simulink model "Rebuilt_AWD"  (R2022a)
settings: Solver=VariableStepAuto  StartTime=0.0  StopTime=100  MaxStep=0.01  RelTol=1e-3
PreLoadFcn:
  | open Vehicle_information
  | run  Vehicle_information
undefined symbols (not defined in the file or in its folder): Rider_mass, sigbuilder_block, Vehicle_mass, wheel_radius
libraries: nesl_utility x30, fl_lib x26, sdl_lib x19
(part 1 of 3)
CloseFcn:
  | clc
  | clear
settings Model: Creator=Aqib Habib  LastModifiedBy=Aqib Habib
settings SolverCC: AlgebraicLoopSolver=LineSearch
settings DebuggingCC: UnconnectedInputMsg=warning  UnconnectedOutputMsg=warning  UnconnectedLineMsg=warning  SFMachineParentedDataDiag=warning
settings SFSimCC: CustomCodeUndefinedFunction=UseInterfaceOnly

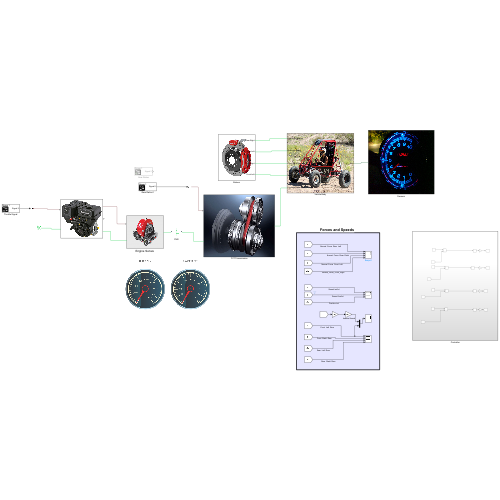
[thumbnail: Simulink's stored preview of the top-level diagram]
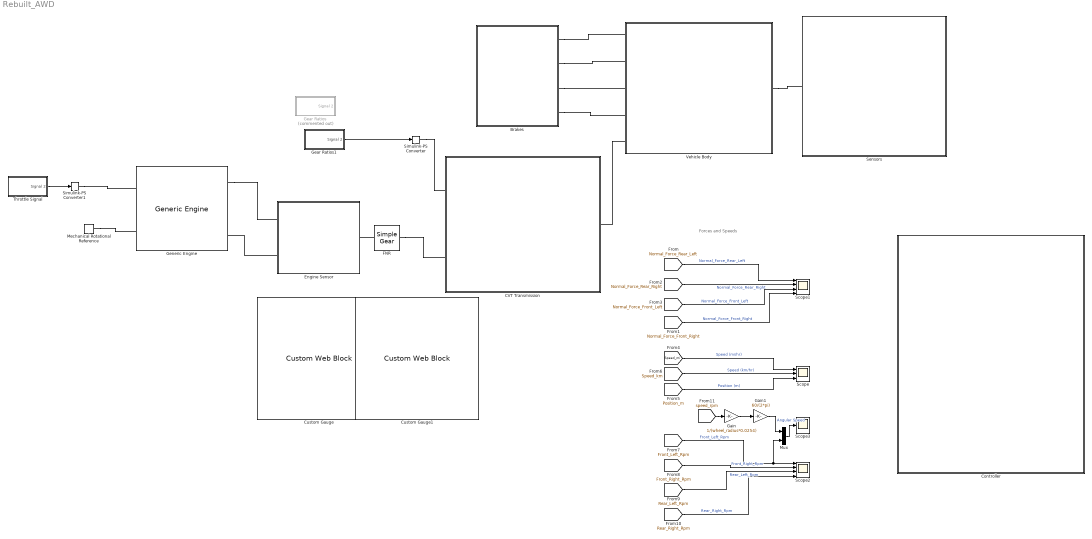
== system Rebuilt_AWD ==
  note: Forces and Speeds
  Brakes : Subsystem
      mask Display: image('brake_kit_140-14883-DR-xl.jpg');
  CVT Transmission : Subsystem
      mask Display: image('CVT-58e526803df78c5162b323c9.jpg');
  "Controller " : Subsystem
  Custom Gauge : CustomWebBlock  Configuration="{\"components\":[{\"name\":\"CircularScaleComponent\",\"settings\":{\"bounds\":{\"max\":100,\"min\":0,\"tickInterval\":\"auto\"},\"direction\":\"cw\",\"flipLimits\":0,\"innerRadius\":0.75,\"internalTickHeightScaleFactor\":1,\"labelColor\":[255,252,199],\"labelFont\":{\"font\":\"Arial\",\"fontSize\":12},\"labelRadius\":0.36,\"labelTransparency\":1,\"minorTickHeightScaleFactor\":0.2,\"needleImage\":{\"size\":[1890,567],\"src\":\"data:image\\/svg+xml;base64,PD94bWwgdmVyc2lvbj0iMS4wIiBlbmNvZGluZz0iVVRGLTgiIHN0YW5kYWxvbmU9Im5vIj8+CjxzdmcKICAgeG1sbnM6ZGM9Imh0dHA6Ly9wdXJsLm9yZy9kYy9lbGVtZW50cy8xLjEvIgogICB4bWxuczpjYz0iaHR0cDovL2NyZWF0aXZlY29tbW9ucy5vcmcvbnMjIgogICB4bWxuczpyZGY9Imh0dHA6Ly93d3cudzMub3JnLzE5OTkvMDIvMjItcmRmLXN5bnRheC1ucyMiCiAgIHhtbG5zOnN2Zz0iaHR0cDovL3d3dy53My5vcmcvMjAwMC9zdmciCiAgIHhtbG5zPSJodHRwOi8vd3d3LnczLm9yZy8yMDAwL3N2ZyIKICAgeG1sbnM6 ...(+4096 chars)\"},\"needleOffset\":[0.14,0],\"needleOrientation\":-45,\"needleRotation\":180,\"needleSize\":{\"height\":0.13,\"width\":0.41},\"outerRadius\":0.9,\"position\":[0.06486742424242424,0.05627705627705628,0.8917748917748918,0.8787878787878788],\"scaleAngle\":270,\"scaleAngleOffset\":135,\"scaleColors\":[],\"scaleColorsSize\":0.2,\"scalePosition\":[0,0,1,1],\"showLabels\":1,\"showMinorTicks\":1,\"showSpanLine\":1,\"showTicks\":1,\"tickColor\":[255,255,200],\"tickTransparency\":1,\"valueBarColor\":[0,114,189],\"valueBarPosition\":[0,0,1,1],\"valueBarSize\":0.2,\"valueBarTransparency\":1}},{\"name\":\"BackgroundImageComponent\",\"settings\":{\"image\":{\"size\":[500,500],\"src\":\"data:image\\/svg+xml;base64,PD94bWwgdmVyc2lvbj0iMS4wIiBlbmNvZGluZz0iVVRGLTgiIHN0YW5kYWxvbmU9Im5vIj8+CjxzdmcKICAgeG1sbnM6ZGM9Imh0dHA6Ly9wdXJsLm9yZy9kYy9lbGVtZW50cy8xLjEvIgogICB4bWxuczpjYz0iaHR0cDovL2NyZWF0aXZlY29tbW9ucy5vcmcvbnMjIgogICB4bWxuczpyZGY9Imh0dHA6Ly93d3cudzMub3JnLzE5OTkvMDIvMjItcmRmLXN5bnRheC1ucyMiCiAgIHhtbG5zOnN2Zz0iaHR0cDovL3d3dy53My5vcmcvMjAwMC9zdmciCiAgIHhtbG5zPSJodHRwOi8vd3d3LnczLm9yZy8yMDAwL3N2ZyIKICAgeG1sbnM6 ...(+9964 chars)\"},\"position\":[0,0,1,1],\"scaleMode\":\"0\"}},{\"name\":\"ForegroundImageComponent\",\"settings\":{\"image\":{\"size\":[0,0],\"src\":\"default\",\"srcOrientation\":[]},\"isForeground\":1,\"position\":[0,0,1,1],\"scaleMode\":\"0\"}}],\"legacySettings\":{\"BackgroundImage\":\"data:image\\/svg+xml;base64,PD94bWwgdmVyc2lvbj0iMS4wIiBlbmNvZGluZz0iVVRGLTgiIHN0YW5kYWxvbmU9Im5vIj8+CjwhLS0gR2VuZXJhdG9yOiBBZG9iZSBJbGx1c3RyYXRvciAxOS4yLjEsIFNWRyBFeHBvcnQgUGx1Zy1JbiAuIFNWRyBWZXJzaW9uOiA2LjAwIEJ1aWxkIDApICAtLT4KCjxzdmcKICAgeG1sbnM6ZGM9Imh0dHA6Ly9wdXJsLm9yZy9kYy9lbGVtZW50cy8xLjEvIgogICB4bWxuczpjYz0iaHR0cDovL2NyZWF0aXZlY29tbW9ucy5vcmcvbnMjIgogICB4bWxuczpyZGY9Imh0dHA6Ly93d3cudzMub3JnLzE5OTkvMDIvMjItcmRmLXN5bnRh ...(+9660 chars)\",\"CenterOffsetX\":\"0\",\"CenterOffsetY\":\"0\",\"GaugeArcColor\":\"#9ec0f7\",\"GaugeArcDefined\":\"true\",\"GaugeArcRadius\":\"0.1358563990074277\",\"GaugeArcRatio\":\"0.8333333333333\",\"GaugeArcRotation\":\"240.5385250290321\",\"GaugeArcStrokeWidth\":\"0.03972965542329953\",\"GaugeArcTransparency\":\"0\",\"GaugeMax\":\"3800\",\"GaugeMin\":\"0\",\"GaugeTickColor\":\"#faf5c8\",\"GaugeTickTransparency\":\"1\",\"GaugeTickVisible\":\"true\",\"GaugeValue\":\"0\",\"NeedleHeight\":\"0.11602152693163792\",\"NeedleImage\":\"data:image\\/svg+xml;base64,PD94bWwgdmVyc2lvbj0iMS4wIiBlbmNvZGluZz0idXRmLTgiPz4KPCEtLSBHZW5lcmF0b3I6IEFkb2JlIElsbHVzdHJhdG9yIDE5LjIuMSwgU1ZHIEV4cG9ydCBQbHVnLUluIC4gU1ZHIFZlcnNpb246IDYuMDAgQnVpbGQgMCkgIC0tPgo8c3ZnIHZlcnNpb249IjEuMSIgeG1sbnM9Imh0dHA6Ly93d3cudzMub3JnLzIwMDAvc3ZnIiB4bWxuczp4bGluaz0iaHR0cDovL3d3dy53My5vcmcvMTk5OS94bGluayIgeD0iMHB4IiB5PSIwcHgiCgkgdmlld0JveD0iMCAwIDIwMCA1MCIgc3R5bGU9ImVuYWJsZS1iYWNrZ3JvdW5kOm5ldyAw ...(+9940 chars)\",\"NeedleInitialRotation\":\"-59.94322499147643\",\"NeedleWidth\":\"0.1911368983686954\",\"NeedleXPos\":\"0.3802298124325669\",\"NeedleYPos\":\"0.48117305677424654\",\"ScaleColorsJSON\":\"[]\",\"ValueArcColor\":\"#1759b0\",\"ValueArcTransparency\":\"1\"},\"settings\":{\"BindingType\":\"signal\",\"backgroundOffset\":0.14,\"backgroundOpacity\":1,\"fixedAspectRatio\":\"on\",\"showBackgroundColor\":0},\"type\":\"CircularGauge\"}"
  Custom Gauge1 : CustomWebBlock  Configuration="{\"components\":[{\"name\":\"CircularScaleComponent\",\"settings\":{\"bounds\":{\"max\":100,\"min\":0,\"tickInterval\":\"auto\"},\"direction\":\"cw\",\"flipLimits\":0,\"innerRadius\":0.75,\"internalTickHeightScaleFactor\":1,\"labelColor\":[255,252,199],\"labelFont\":{\"font\":\"Arial\",\"fontSize\":12},\"labelRadius\":0.36,\"labelTransparency\":1,\"minorTickHeightScaleFactor\":0.2,\"needleImage\":{\"size\":[1890,567],\"src\":\"data:image\\/svg+xml;base64,PD94bWwgdmVyc2lvbj0iMS4wIiBlbmNvZGluZz0iVVRGLTgiIHN0YW5kYWxvbmU9Im5vIj8+CjxzdmcKICAgeG1sbnM6ZGM9Imh0dHA6Ly9wdXJsLm9yZy9kYy9lbGVtZW50cy8xLjEvIgogICB4bWxuczpjYz0iaHR0cDovL2NyZWF0aXZlY29tbW9ucy5vcmcvbnMjIgogICB4bWxuczpyZGY9Imh0dHA6Ly93d3cudzMub3JnLzE5OTkvMDIvMjItcmRmLXN5bnRheC1ucyMiCiAgIHhtbG5zOnN2Zz0iaHR0cDovL3d3dy53My5vcmcvMjAwMC9zdmciCiAgIHhtbG5zPSJodHRwOi8vd3d3LnczLm9yZy8yMDAwL3N2ZyIKICAgeG1sbnM6 ...(+4096 chars)\"},\"needleOffset\":[0.14,0],\"needleOrientation\":-45,\"needleRotation\":180,\"needleSize\":{\"height\":0.13,\"width\":0.41},\"outerRadius\":0.9,\"position\":[0.06486742424242424,0.05627705627705628,0.8917748917748918,0.8787878787878788],\"scaleAngle\":270,\"scaleAngleOffset\":135,\"scaleColors\":[],\"scaleColorsSize\":0.2,\"scalePosition\":[0,0,1,1],\"showLabels\":1,\"showMinorTicks\":1,\"showSpanLine\":1,\"showTicks\":1,\"tickColor\":[255,255,200],\"tickTransparency\":1,\"valueBarColor\":[0,114,189],\"valueBarPosition\":[0,0,1,1],\"valueBarSize\":0.2,\"valueBarTransparency\":1}},{\"name\":\"BackgroundImageComponent\",\"settings\":{\"image\":{\"size\":[500,500],\"src\":\"data:image\\/svg+xml;base64,PD94bWwgdmVyc2lvbj0iMS4wIiBlbmNvZGluZz0iVVRGLTgiIHN0YW5kYWxvbmU9Im5vIj8+CjxzdmcKICAgeG1sbnM6ZGM9Imh0dHA6Ly9wdXJsLm9yZy9kYy9lbGVtZW50cy8xLjEvIgogICB4bWxuczpjYz0iaHR0cDovL2NyZWF0aXZlY29tbW9ucy5vcmcvbnMjIgogICB4bWxuczpyZGY9Imh0dHA6Ly93d3cudzMub3JnLzE5OTkvMDIvMjItcmRmLXN5bnRheC1ucyMiCiAgIHhtbG5zOnN2Zz0iaHR0cDovL3d3dy53My5vcmcvMjAwMC9zdmciCiAgIHhtbG5zPSJodHRwOi8vd3d3LnczLm9yZy8yMDAwL3N2ZyIKICAgeG1sbnM6 ...(+9964 chars)\"},\"position\":[0,0,1,1],\"scaleMode\":\"0\"}},{\"name\":\"ForegroundImageComponent\",\"settings\":{\"image\":{\"size\":[0,0],\"src\":\"default\",\"srcOrientation\":[]},\"isForeground\":1,\"position\":[0,0,1,1],\"scaleMode\":\"0\"}}],\"legacySettings\":{\"BackgroundImage\":\"data:image\\/svg+xml;base64,PD94bWwgdmVyc2lvbj0iMS4wIiBlbmNvZGluZz0iVVRGLTgiIHN0YW5kYWxvbmU9Im5vIj8+CjwhLS0gR2VuZXJhdG9yOiBBZG9iZSBJbGx1c3RyYXRvciAxOS4yLjEsIFNWRyBFeHBvcnQgUGx1Zy1JbiAuIFNWRyBWZXJzaW9uOiA2LjAwIEJ1aWxkIDApICAtLT4KCjxzdmcKICAgeG1sbnM6ZGM9Imh0dHA6Ly9wdXJsLm9yZy9kYy9lbGVtZW50cy8xLjEvIgogICB4bWxuczpjYz0iaHR0cDovL2NyZWF0aXZlY29tbW9ucy5vcmcvbnMjIgogICB4bWxuczpyZGY9Imh0dHA6Ly93d3cudzMub3JnLzE5OTkvMDIvMjItcmRmLXN5bnRh ...(+9660 chars)\",\"CenterOffsetX\":\"0\",\"CenterOffsetY\":\"0\",\"GaugeArcColor\":\"#9ec0f7\",\"GaugeArcDefined\":\"true\",\"GaugeArcRadius\":\"0.1358563990074277\",\"GaugeArcRatio\":\"0.8333333333333\",\"GaugeArcRotation\":\"240.5385250290321\",\"GaugeArcStrokeWidth\":\"0.03972965542329953\",\"GaugeArcTransparency\":\"0\",\"GaugeMax\":\"100\",\"GaugeMin\":\"0\",\"GaugeTickColor\":\"#faf5c8\",\"GaugeTickTransparency\":\"1\",\"GaugeTickVisible\":\"true\",\"GaugeValue\":\"0\",\"NeedleHeight\":\"0.11602152693163792\",\"NeedleImage\":\"data:image\\/svg+xml;base64,PD94bWwgdmVyc2lvbj0iMS4wIiBlbmNvZGluZz0idXRmLTgiPz4KPCEtLSBHZW5lcmF0b3I6IEFkb2JlIElsbHVzdHJhdG9yIDE5LjIuMSwgU1ZHIEV4cG9ydCBQbHVnLUluIC4gU1ZHIFZlcnNpb246IDYuMDAgQnVpbGQgMCkgIC0tPgo8c3ZnIHZlcnNpb249IjEuMSIgeG1sbnM9Imh0dHA6Ly93d3cudzMub3JnLzIwMDAvc3ZnIiB4bWxuczp4bGluaz0iaHR0cDovL3d3dy53My5vcmcvMTk5OS94bGluayIgeD0iMHB4IiB5PSIwcHgiCgkgdmlld0JveD0iMCAwIDIwMCA1MCIgc3R5bGU9ImVuYWJsZS1iYWNrZ3JvdW5kOm5ldyAw ...(+9940 chars)\",\"NeedleInitialRotation\":\"-59.94322499147643\",\"NeedleWidth\":\"0.1911368983686954\",\"NeedleXPos\":\"0.3802298124325669\",\"NeedleYPos\":\"0.48117305677424654\",\"ScaleColorsJSON\":\"[]\",\"ValueArcColor\":\"#1759b0\",\"ValueArcTransparency\":\"1\"},\"settings\":{\"BindingType\":\"signal\",\"backgroundOffset\":0.14,\"backgroundOpacity\":1,\"fixedAspectRatio\":\"on\",\"showBackgroundColor\":0},\"type\":\"CircularGauge\"}"
  Engine Sensor : Subsystem
      mask Display: image('eddy-current-engine-dynamometer_cat-1024x878.jpg');
  FNR : sdl_lib/Gears/Simple Gear  ratio=4  rotation_direction=3-2*(1)  friction_model=sdl.enum.gear_efficiencies_load.off  T_noload=0.1 N*m  T_nom=5 N*m  efficiency_nom=0.8  efficiency=0.8  temperature_TLU=[280, 300, 320] K  load_TLU=[1, 5, 10] N*m  efficiency_TLU=[.95, .9, .85]  efficiency_TLU2=[.85, .8, .75; .95, .9, .85; .85, .8, .7]  w_thr=0.01 rad/s  pwr_thr=0.001 W  backlash_model=sdl.enum.backlashModel.Off  backlash_distance=1e-3 mm  x0=0 mm  r_base=0.1 m  hardstop_model=simscape.enum.hardstop.smooth  transition=1e-4 mm  backlash_stiffness=1e7 N/m  backlash_damping=1e6 N*s/m  e=0  v_tol=0.001 m/s  mu_visc=[0, 0] N*m/(rad/s)  enable_faults=simscape.enum.onoff.off  efficiency_fault=0.05  external_fault=simscape.enum.onoff.off  temporal_fault=simscape.enum.onoff.off  fault_time=5 s  fault_angles=pi / 12 rad  report_fault=(1)-1  thermal_mass=50 J/K  temperature_specify=off  temperature_priority=High  temperature=300 K  temperature_nominal_specify=off  temperature_nominal_unit=K  temperature_nominal_value=1  x_backlash_specify=off  x_backlash_priority=None  x_backlash=0 mm  x_backlash_nominal_specify=off  x_backlash_nominal_unit=mm  x_backlash_nominal_value=1  f_hardstop_specify=off  f_hardstop_priority=None  f_hardstop=0 N  f_hardstop_nominal_specify=off  f_hardstop_nominal_unit=N  f_hardstop_nominal_value=1  v_backlash_specify=off  v_backlash_priority=None  v_backlash=0 m/s  v_backlash_nominal_specify=off  v_backlash_nominal_unit=m/s  v_backlash_nominal_value=1
  Gain : Gain  Gain=1/(wheel_radius*0.0254)
  Gain1 : Gain  Gain=60/(2*pi)
  Gear Ratios : Subsystem  Tag=STV Subsys  Commented=on  LoadFcn=sigbuilder_block('load');  StartFcn=sigbuilder_block('start');  StopFcn=sigbuilder_block('stop');  ClipboardFcn=sigbuilder_block('clipboard');  mask(Sigbuilder block){tuvar=[0:10]}
      mask help: Simulink:masks:SigbuilderBlock_MD
      mask init:
      | if ~strcmp(get_param(bdroot(gcbh),'SimulationStatus'),'stopped') tuvar = sigbuilder_block('maskInit'); end
      settings: CopyFcn=sigbuilder_block('copy');  DeleteFcn=sigbuilder_block('delete');  ModelCloseFcn=sigbuilder_block('modelClose');  PreSaveFcn=sigbuilder_block('preSave');  PauseFcn=sigbuilder_block('pause');  ContinueFcn=sigbuilder_block('continue');  NameChangeFcn=sigbuilder_block('namechange');  OpenFcn=sigbuilder_block('open',[6 30 1428 681.75 ]);  CloseFcn=sigbuilder_block('close');
      mask Display: plot(0, 0, 100, 100,[2, 2, 32, 32, 2], [68, 8, 8, 68, 68],[32, 2], [38, 38], [32, 19, 2],[53, 60, 44], [32, 17, 17, 2],[16, 16, 31, 31]);txt = getActiveGroup(gcbh);text(2, 100, txt,'verticalAlignment', 'top');
  Gear Ratios1 : Subsystem  Tag=STV Subsys  LoadFcn=sigbuilder_block('load');  StartFcn=sigbuilder_block('start');  StopFcn=sigbuilder_block('stop');  ClipboardFcn=sigbuilder_block('clipboard');  mask(Sigbuilder block){tuvar=[0:10]}
      mask help: Simulink:masks:SigbuilderBlock_MD
      mask init:
      | if ~strcmp(get_param(bdroot(gcbh),'SimulationStatus'),'stopped') tuvar = sigbuilder_block('maskInit'); end
      settings: CopyFcn=sigbuilder_block('copy');  DeleteFcn=sigbuilder_block('delete');  ModelCloseFcn=sigbuilder_block('modelClose');  PreSaveFcn=sigbuilder_block('preSave');  PauseFcn=sigbuilder_block('pause');  ContinueFcn=sigbuilder_block('continue');  NameChangeFcn=sigbuilder_block('namechange');  OpenFcn=sigbuilder_block('open',[6 30 1428 681.75 ]);  CloseFcn=sigbuilder_block('close');
      mask Display: plot(0, 0, 100, 100,[2, 2, 32, 32, 2], [68, 8, 8, 68, 68],[32, 2], [38, 38], [32, 19, 2],[53, 60, 44], [32, 17, 17, 2],[16, 16, 31, 31]);txt = getActiveGroup(gcbh);text(2, 100, txt,'verticalAlignment', 'top');
  Generic Engine : sdl_lib/Engines & Motors/Generic Engine  model_parameterization=3  engine_type=1  P_max=150 kW  w_P_max=4500 rpm  w_max=6000 rpm  w_min=500 rpm  w_tab=RPM rpm  trq_tab=[380, 380, 380, 380, 350, 280, 200, 80] N*m  pwr_tab=POWER HP_DIN  interp_method=simscape.enum.interpolation.smooth  model_inertia=1  inertia=5 kg*m^2  initial_velocity=2200 rpm  model_time_constant=0  time_constant=0.2 s  T0=0  w_thr=100 rpm  fc_model=0  fc_per_rev=25 mg/rev  fc_w_tab=[1000, 2000, 3000, 4000, 5000, 6000] rpm  fc_trq_tab=[0, 80, 160, 200, 240, 320, 360, 400] N*m  fc_tab=[.5, .9, 1.4, 1.6, 1.9, 2.7, 3.4, 4.4; 1, 1.7, 2.7, 3.1, 3.6, 5, 6, 7.4; 1.4, 2.7, 4, 4.8, 5.6, 7.5, 8.5, 10.5; 2, 3.6, 5.8, 6.7, 8, 10.4, 11.7, 13.3; 2.5, 4.8, 7.9, 9.4, 10.8, 14, 16.2, 18.6; 3.1, 6, 10.3, 11.9, 13.8, 18.4, 22, 26.5] g/s  bmep_tab=[0, 250, 500, 625, 750, 1000, 1150, 1250] kPa  bsfc_tab=[410, 380, 300, 280, 270, 290, 320, 380; 410, 370, 290, 270, 260, 270, 285, 320; 415, 380, 290, 275, 265, 270, 270, 300; 420, 390, 310, 290, 285, 280, 280, 285; 430, 410, 340, 320, 310, 300, 310, 320; 450, 430, 370, 340, 330, 330, 350, 380] g/hr/kW  fc_interp_method=simscape.enum.interpolation.linear  idle_speed=0  idle_speed_reference=3600 rpm  tau_controller=1 s  idle_w_thr=1 rpm  redline=0  redline_speed=5000 rpm  tau_redline=1 s  redline_w_thr=1 rpm  displaced_volume=400 cm^3  rev_per_cycle=2  mask(Generic Engine){}
      settings: SourceProductBaseCode=LD  InternalSimscapePortConfiguration="{\"Bottom\":[],\"Left\":[{\"id\":\"T\",\"label\":\"T\",\"type\":\"input\"},{\"id\":\"B\",\"label\":\"B\",\"type\":\"foundation.mechanical.rotational.rotational\"}],\"Right\":[{\"id\":\"P\",\"label\":\"P\",\"type\":\"output\"},{\"id\":\"FC\",\"label\":\"FC\",\"type\":\"output\"},{\"id\":\"F\",\"label\":\"F\",\"type\":\"foundation.mechanical.rotational.rotational\"}],\"Top\":[]}"
      mask Display: image('10.0hp_updated.jpg');
  Mechanical Rotational Reference : fl_lib/Mechanical/Rotational Elements/Mechanical Rotational Reference
      settings: SourceProductBaseCode=PW,SS,VE
  Mux : Mux  Inputs=2
  Scope : Scope  NumInputPorts=3
  Scope1 : Scope  NumInputPorts=4
  Scope2 : Scope  NumInputPorts=4
  Scope3 : Scope
  Sensors : Subsystem
      mask Display: image('wp6910276.jpg');
  Simulink-PS Converter : nesl_utility/Simulink-PS Converter  PhysicalDomain=network_engine_domain  SubClassName=ps_input  LeftPortType=input  RightPortType=output  PseudoPeriodic=off  Frequencies=[]  NoiseDistribution=none  NoiseParameters=[]  Unit=1  AffineConversion=off  FilteringAndDerivatives=provide  SimscapeFilterOrder=1  InputFilterTimeConstant=0.001  UdotUserProvided=0
      settings: SourceProductBaseCode=SS,PW,VE
  Simulink-PS Converter1 : nesl_utility/Simulink-PS Converter  PhysicalDomain=network_engine_domain  SubClassName=ps_input  LeftPortType=input  RightPortType=output  PseudoPeriodic=off  Frequencies=[]  NoiseDistribution=none  NoiseParameters=[]  Unit=1  AffineConversion=off  FilteringAndDerivatives=provide  SimscapeFilterOrder=1  InputFilterTimeConstant=0.001  UdotUserProvided=0
      settings: SourceProductBaseCode=SS,PW,VE
  Throttle Signal : Subsystem  Tag=STV Subsys  LoadFcn=sigbuilder_block('load');  StartFcn=sigbuilder_block('start');  StopFcn=sigbuilder_block('stop');  ClipboardFcn=sigbuilder_block('clipboard');  mask(Sigbuilder block){tuvar=[0:10]}
      mask help: Simulink:masks:SigbuilderBlock_MD
      mask init:
      | if ~strcmp(get_param(bdroot(gcbh),'SimulationStatus'),'stopped') tuvar = sigbuilder_block('maskInit'); end
      settings: CopyFcn=sigbuilder_block('copy');  DeleteFcn=sigbuilder_block('delete');  ModelCloseFcn=sigbuilder_block('modelClose');  PreSaveFcn=sigbuilder_block('preSave');  PauseFcn=sigbuilder_block('pause');  ContinueFcn=sigbuilder_block('continue');  NameChangeFcn=sigbuilder_block('namechange');  OpenFcn=sigbuilder_block('open',[6 30 1428 681.75 ]);  CloseFcn=sigbuilder_block('close');
      mask Display: plot(0, 0, 100, 100,[2, 2, 32, 32, 2], [68, 8, 8, 68, 68],[32, 2], [38, 38], [32, 19, 2],[53, 60, 44], [32, 17, 17, 2],[16, 16, 31, 31]);txt = getActiveGroup(gcbh);text(2, 100, txt,'verticalAlignment', 'top');
  Vehicle Body : Subsystem
      mask Display: image('Mini_Baja.jpg');
  wires:
  Throttle Signal/1(Signal 2) -> Simulink-PS Converter1/1
  [Normal_Force_Rear_Left] -> Scope1/1  "Normal_Force_Rear_Left"
  [Normal_Force_Front_Right] -> Scope1/4  "Normal_Force_Front_Right"
  [Normal_Force_Rear_Right] -> Scope1/2  "Normal_Force_Rear_Right"
  [Normal_Force_Front_Left] -> Scope1/3  "Normal_Force_Front_Left"
  [Speed_mi] -> Scope/1  "Speed (mi/hr)"
  [Position_m] -> Scope/3  "Position (m)"
  [Speed_km] -> Scope/2  "Speed (km/hr)"
  [Front_Left_Rpm] -> Mux/2, Scope2/1  "Front_Left_Rpm"
  [Front_Right_Rpm] -> Scope2/2  "Front_Right_Rpm"
  [Rear_Left_Rpm] -> Scope2/3  "Rear_Left_Rpm"
  [Rear_Right_Rpm] -> Scope2/4  "Rear_Right_Rpm"
  [speed_rpm] -> Gain/1
  Gain/1 -> Gain1/1
  Gear Ratios1/1(Signal 2) -> Simulink-PS Converter/1
  Gain1/1 -> Mux/1  "Angular Speed"
  Mux/1 -> Scope3/1
  connections:
  Simulink-PS Converter/RConn1 -- CVT Transmission/LConn1
  Simulink-PS Converter1/RConn1 -- Generic Engine/LConn1
  Mechanical Rotational Reference/LConn1 -- Generic Engine/LConn2
  Engine Sensor/LConn2 -- Generic Engine/RConn3
  Vehicle Body/RConn1 -- Sensors/LConn1
  Brakes/RConn1 -- Vehicle Body/LConn1
  Brakes/RConn2 -- Vehicle Body/LConn2
  Brakes/RConn3 -- Vehicle Body/LConn3
  Brakes/RConn4 -- Vehicle Body/LConn4
  Vehicle Body/LConn5 -- CVT Transmission/RConn1
  FNR/LConn1 -- Engine Sensor/RConn1
  FNR/RConn1 -- CVT Transmission/LConn2
  Generic Engine/RConn1 -- Engine Sensor/LConn1
